simulink library "DoorRlsReq"  (R2022a)
settings: Solver=VariableStepAuto  StartTime=0.0  StopTime=10.0  RelTol=1e-3
settings Model: Creator=DELL  LastModifiedBy=liyun

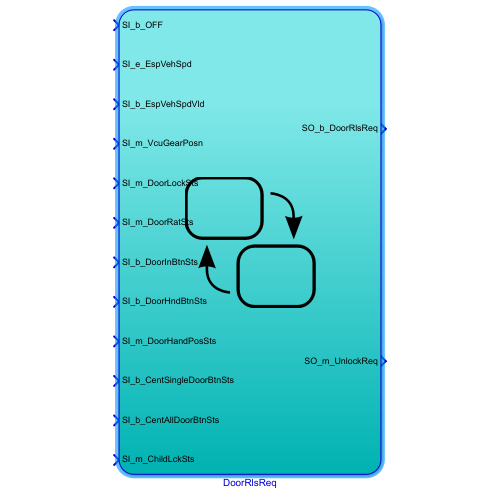
[thumbnail: Simulink's stored preview of the top-level diagram]
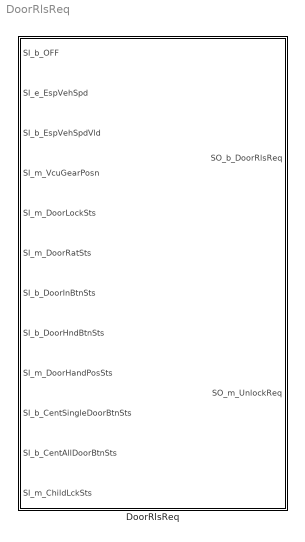
== system DoorRlsReq ==
  DoorRlsReq : Stateflow chart  TreatAsAtomicUnit=on

== stateflow chart DoorRlsReq/DoorRlsReq ==
  state DoorInBtn [parallel]
    settings: executionOrder=1
    state SwValid [parallel]
      settings: executionOrder=1
      state Idle
        en:
        SL_b_DoorInBtnValid = 0;
      state Once
      state Twice
        en:
        SL_b_DoorInBtnValid = 1;
      (default) -> DoorInBtn.SwValid.Idle
      DoorInBtn.SwValid.Idle -> Once : [hasChangedTo(SI_b_DoorInBtnSts, 1)]
      Once -> Twice [order 1] : [hasChangedTo(SI_b_DoorInBtnSts, 1)]
      Once -> DoorInBtn.SwValid.Idle [order 2] : [after(200, tick)]
      Twice -> DoorInBtn.SwValid.Idle : [after(3, tick)]
    state RlsReq [parallel]
      settings: executionOrder=2
      state Idle
      state Trigger
        state DoorLock
          state UnlockReq
            en:
            SO_m_UnlockReq = Unlock_Req;
            on at(5, tick):
            SO_m_UnlockReq = Unlock_Idle;
          state UnlockSuccess
          state UnlockFail
          (default) -> DoorInBtn.RlsReq.Trigger.DoorLock.UnlockReq
          DoorInBtn.RlsReq.Trigger.DoorLock.UnlockReq -> DoorInBtn.RlsReq.Trigger.DoorLock.UnlockFail [order 2] : [after(50, tick) && ...
              | SI_m_DoorLockSts == Door_Lock]
          DoorInBtn.RlsReq.Trigger.DoorLock.UnlockReq -> UnlockSuccess [order 1] : [SI_m_DoorLockSts == Door_Unlock]
        state Release
          en:
          SO_b_DoorRlsReq = 1;
        state DoorUnlock
        state Error
        (default) -> DoorInBtn.RlsReq.Trigger.DoorLock [order 1] : [SI_m_DoorLockSts == Door_Lock]
        (default) -> DoorInBtn.RlsReq.Trigger.DoorUnlock [order 2] : [SI_m_DoorLockSts == Door_Unlock]
        DoorInBtn.RlsReq.Trigger.DoorUnlock -> DoorInBtn.RlsReq.Trigger.Release : [SI_m_DoorRatSts != Rat_Unlock]
        (default) -> DoorInBtn.RlsReq.Trigger.Error [order 3]
        UnlockSuccess -> DoorInBtn.RlsReq.Trigger.Release : [SI_m_DoorRatSts != Rat_Unlock]
      (default) -> DoorInBtn.RlsReq.Idle
      DoorInBtn.RlsReq.Idle -> DoorInBtn.RlsReq.Trigger : [(SI_e_EspVehSpd < 5 && SI_b_EspVehSpdVld == 0) && ...
          | SI_m_ChildLckSts == Child_Unlock && ...
          | hasChangedTo(SL_b_DoorInBtnValid, 1)]
      DoorInBtn.RlsReq.Trigger -> DoorInBtn.RlsReq.Idle : [(SI_e_EspVehSpd >= 5 && SI_b_EspVehSpdVld == 0) || ...
          | SI_m_ChildLckSts != Child_Unlock || ...
          | (SI_m_DoorLockSts == Door_Unlock && ...
          | SI_m_DoorRatSts == Rat_Unlock)]
      DoorInBtn.RlsReq.Trigger.Release -> (junction 173) : [after(5, tick)]
          | {SO_b_DoorRlsReq = 0;}
      DoorInBtn.RlsReq.Trigger.Error -> DoorInBtn.RlsReq.Idle
      (junction 173) -> DoorInBtn.RlsReq.Idle
      DoorInBtn.RlsReq.Trigger.DoorLock.UnlockFail -> DoorInBtn.RlsReq.Idle
  state DoorHndBtn [parallel]
    settings: executionOrder=2
    state SwValid [parallel]
      settings: executionOrder=2
      state Idle
        en,du:
        SL_b_DoorHndBtnValid = SI_b_DoorHndBtnSts;
      (default) -> DoorHndBtn.SwValid.Idle
    state RlsReq [parallel]
      settings: executionOrder=1
      state Idle
      state Trigger
        state Release
          en:
          SO_b_DoorRlsReq = 1;
        state DoorUnlock
        (default) -> DoorHndBtn.RlsReq.Trigger.DoorUnlock
        DoorHndBtn.RlsReq.Trigger.DoorUnlock -> DoorHndBtn.RlsReq.Trigger.Release : [SI_m_DoorRatSts != Rat_Unlock]
      (default) -> DoorHndBtn.RlsReq.Idle
      DoorHndBtn.RlsReq.Idle -> DoorHndBtn.RlsReq.Trigger : [(SI_e_EspVehSpd < 5 && SI_b_EspVehSpdVld == 0) && ...
          | SI_m_DoorLockSts == Door_Unlock && ...
          | hasChangedTo(SL_b_DoorHndBtnValid, 1)]
      DoorHndBtn.RlsReq.Trigger -> DoorHndBtn.RlsReq.Idle : [(SI_e_EspVehSpd >= 5 && SI_b_EspVehSpdVld == 0) || ...
          | SI_m_DoorLockSts != Door_Unlock || ...
          | SI_m_DoorRatSts == Rat_Unlock]
      DoorHndBtn.RlsReq.Trigger.Release -> (junction 265) : [after(5,tick)]
          | {SO_b_DoorRlsReq = 0;}
      (junction 265) -> DoorHndBtn.RlsReq.Idle
  state CentDoorBtn [parallel] [commented out]
    state SwValid [parallel] [commented out]
      state Idle [commented out]
        en,du:
        SL_b_CentSingleDoorBtnValid = SI_b_CentSingleDoorBtnSts;
        SL_b_CentAllDoorBtnValid = SI_b_CentAllDoorBtnSts;
      (default) -> CentDoorBtn.SwValid.Idle [commented out]
    state DoorCentral [parallel] [commented out]
      state Idle [commented out]
      state Trigger [commented out]
        state DoorLock [commented out]
          state UnlockReq [commented out]
            en:
            SO_m_UnlockReq = Unlock_Req;
            on at(5, tick):
            SO_m_UnlockReq = Unlock_Idle;
          state UnlockSucess [commented out]
          state UnlockFail [commented out]
          (default) -> CentDoorBtn.DoorCentral.Trigger.DoorLock.UnlockReq [commented out]
          CentDoorBtn.DoorCentral.Trigger.DoorLock.UnlockReq -> CentDoorBtn.DoorCentral.Trigger.DoorLock.UnlockFail [commented out] : [after(50, tick) && ...
              | SI_m_DoorLockSts == Door_Lock]
          CentDoorBtn.DoorCentral.Trigger.DoorLock.UnlockReq -> UnlockSucess [commented out] : [SI_m_DoorLockSts == Door_Unlock]
        state RELEASE [commented out]
          en:
          SO_b_DoorRlsReq = 1;
        state DoorUnlock [commented out]
        state Error [commented out]
        (default) -> CentDoorBtn.DoorCentral.Trigger.DoorLock [commented out] : [SI_m_DoorLockSts == Door_Lock]
        (default) -> CentDoorBtn.DoorCentral.Trigger.DoorUnlock [commented out] : [SI_m_DoorLockSts == Door_Unlock]
        CentDoorBtn.DoorCentral.Trigger.DoorUnlock -> RELEASE [commented out] : [SI_m_DoorRatSts != Rat_Unlock]
        (default) -> CentDoorBtn.DoorCentral.Trigger.Error [commented out]
        UnlockSucess -> RELEASE [commented out] : [SI_m_DoorRatSts != Rat_Unlock]
      (default) -> CentDoorBtn.DoorCentral.Idle [commented out]
      CentDoorBtn.DoorCentral.Idle -> CentDoorBtn.DoorCentral.Trigger [commented out] : [!SI_b_OFF &&...
          | ((SI_e_EspVehSpd <= 0 && SI_b_EspVehSpdVld == 0) ||...
          | SI_m_VcuGearPosn == Gear_P) &&...
          | (hasChangedTo(SL_b_CentSingleDoorBtnValid, 1) ||...
          | hasChangedTo(SL_b_CentAllDoorBtnValid, 1))]
      CentDoorBtn.DoorCentral.Trigger -> CentDoorBtn.DoorCentral.Idle [commented out] : [SI_b_OFF ||...
          | ((SI_e_EspVehSpd >= 1 && SI_b_EspVehSpdVld == 0) &&...
          | SI_m_VcuGearPosn != Gear_P) ||...
          | (SI_m_DoorLockSts == Door_Unlock && ...
          | SI_m_DoorRatSts == Rat_Unlock)]
      RELEASE -> (junction 82) [commented out] : [after(5,tick)]
          | {SO_b_DoorRlsReq = 0;}
      CentDoorBtn.DoorCentral.Trigger.Error -> CentDoorBtn.DoorCentral.Idle [commented out]
      (junction 82) -> CentDoorBtn.DoorCentral.Idle [commented out]
      CentDoorBtn.DoorCentral.Trigger.DoorLock.UnlockFail -> CentDoorBtn.DoorCentral.Idle [commented out]
  state SwValid [parallel] [commented out]
    state Idle [commented out]
      en:
      SL_b_DoorHndBtnValid = 0;
    state Press [commented out]
    state Release [commented out]
      en:
      SL_b_DoorHndBtnValid = 1;
    (default) -> SwValid.Idle [commented out]
    SwValid.Idle -> Press [commented out] : [hasChangedTo(SI_b_DoorHndBtnSts, 1)]
    Press -> SwValid.Release [commented out] : [hasChangedTo(SI_b_DoorHndBtnSts, 0)]
    Press -> SwValid.Idle [commented out] : [after(100, tick)]
    SwValid.Release -> SwValid.Idle [commented out] : [after(3, tick)]
  data: SI_b_OFF input boolean; SI_e_EspVehSpd input uint8; SI_b_EspVehSpdVld input boolean; SI_m_VcuGearPosn input Enum: Gear_Posn_E; SO_b_DoorRlsReq output boolean; SI_m_DoorLockSts input Enum: Door_Sts_E; SI_m_DoorRatSts input Enum: Rat_Sts_E; SO_m_UnlockReq output Enum: Unlock_Req_E; SI_b_DoorInBtnSts input boolean; SI_b_DoorHndBtnSts input boolean; SI_m_DoorHandPosSts input Enum: HndPos_Sts_E; SI_b_CentSingleDoorBtnSts input boolean; SI_b_CentAllDoorBtnSts input boolean; SL_b_DoorInBtnValid local boolean; SL_b_CentSingleDoorBtnValid local boolean; SL_b_CentAllDoorBtnValid local boolean; SI_m_ChildLckSts input Enum: Child_Sts_E; SL_b_DoorHndPullValid local boolean; SL_b_DoorHndBtnValid local boolean
